simulink model "HDLTxRx"  (R2024a)
settings: Solver=FixedStepDiscrete  StartTime=0.0  StopTime=stopTime  RelTol=1e-3
values from neighbouring files (symbols this model uses):
  msgQtty = length(msgIn)    [testTxRx.m]
  pWords = [pWords binl2str(pBits{i})]    [testTxRx.m]
undefined symbols (not defined in the file or in its folder): CONST
libraries: dspsrcs4 x7, HDL_ieee_8021513 x6, hdlsllib x3
settings Model: DataTypeOverride=Off  SimulationMode=accelerator  Creator=cotti  LastModifiedBy=cotti
settings OptimizationCC: BlockReduction=off  ConditionallyExecuteInputs=off  DefaultParameterBehavior=Inlined  InheritOutputTypeSmallerThanSingle=on
settings DebuggingCC: ArtificialAlgebraicLoopMsg=error  SingleTaskRateTransMsg=error
settings HardwareCC: ProdBitPerPointer=32  ProdBitPerSizeT=32  ProdBitPerPtrDiffT=32  ProdLargestAtomicFloat=None  ProdIntDivRoundTo=Undefined  ProdEndianess=Unspecified  ProdWordSize=32  ProdHWDeviceType=ASIC/FPGA->ASIC/FPGA  TargetBitPerLong=64  TargetBitPerPointer=64  TargetBitPerSizeT=64  TargetBitPerPtrDiffT=64  TargetLongLongMode=on  TargetIntDivRoundTo=Zero  TargetEndianess=LittleEndian  TargetWordSize=64  TargetHWDeviceType=Custom Processor->MATLAB Host Computer  ProdEqTarget=off

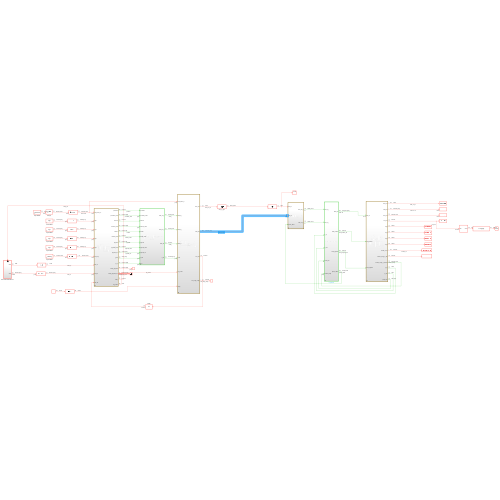
[thumbnail: Simulink's stored preview of the top-level diagram]
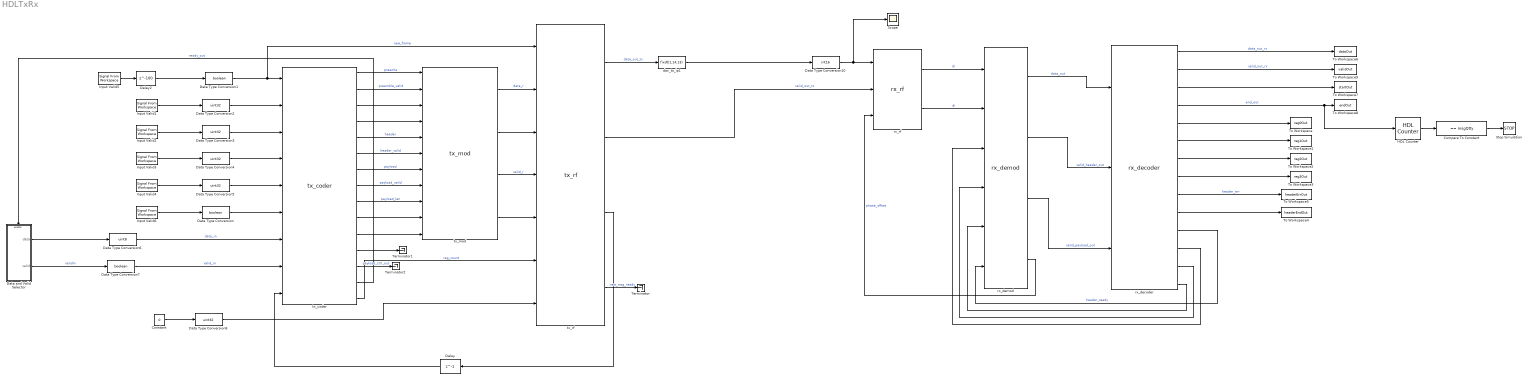
== system HDLTxRx ==
  Compare To Constant : hdlsllib/Logic and Bit Operations/Compare To Constant  relop===  const=msgQtty  OutDataTypeStr=boolean
  Constant : Constant  Value=0  OutDataTypeStr=uint32  SampleTime=-1
  Data Type Conversion : DataTypeConversion  OutDataTypeStr=boolean  SaturateOnIntegerOverflow=off  RndMeth=Floor
  Data Type Conversion1 : DataTypeConversion  OutDataTypeStr=boolean  SaturateOnIntegerOverflow=off  RndMeth=Floor
  Data Type Conversion10 : DataTypeConversion  OutDataTypeStr=int16  ConvertRealWorld=Stored Integer (SI)  SaturateOnIntegerOverflow=off  RndMeth=Floor
  Data Type Conversion{2..5,8} (5 alike) : DataTypeConversion  OutDataTypeStr=uint32  SaturateOnIntegerOverflow=off  RndMeth=Floor
  Data Type Conversion6 : DataTypeConversion  OutDataTypeStr=uint8  SaturateOnIntegerOverflow=off  RndMeth=Floor
  Data Type Conversion7 : DataTypeConversion  OutDataTypeStr=boolean  SaturateOnIntegerOverflow=off  RndMeth=Floor
  Data and Valid Selector : Subsystem  TreatAsAtomicUnit=on
  Delay : Delay  DelayLength=1  InitialCondition=0  UseCircularBuffer=on
  Delay2 : Delay  DelayLength=100  InitialCondition=0  UseCircularBuffer=on
  HDL Counter : hdlsllib/Sources/HDL Counter  CountType=Free running  CountInit=0  CountStep=1  CountMax=25  CountFromType=Initial value  CountFrom=0  CountResetPort=off  CountLoadPort=off  CountEnbPort=on  CountDirPort=off  CountHitOutputPort=off  CountDataType=Unsigned  CountWordLen=32  CountFracLen=0  CountSampTime=1
  Input Valid1 : dspsrcs4/Signal From Workspace  X=reg0  Ts=1/CONST.fs  nsamps=1  OutputAfterFinalValue=Setting to zero  ignoreOrWarnInputAndFrameLengths=off  OutputFrames=off
  Input Valid2 : dspsrcs4/Signal From Workspace  X=reg1  Ts=1/CONST.fs  nsamps=1  OutputAfterFinalValue=Setting to zero  ignoreOrWarnInputAndFrameLengths=off  OutputFrames=off
  Input Valid3 : dspsrcs4/Signal From Workspace  X=reg2  Ts=1/CONST.fs  nsamps=1  OutputAfterFinalValue=Setting to zero  ignoreOrWarnInputAndFrameLengths=off  OutputFrames=off
  Input Valid4 : dspsrcs4/Signal From Workspace  X=reg3  Ts=1/CONST.fs  nsamps=1  OutputAfterFinalValue=Setting to zero  ignoreOrWarnInputAndFrameLengths=off  OutputFrames=off
  Input Valid5 : dspsrcs4/Signal From Workspace  X=newFrame  Ts=1/CONST.fs  nsamps=1  OutputAfterFinalValue=Setting to zero  ignoreOrWarnInputAndFrameLengths=off  OutputFrames=off
  Input Valid6 : dspsrcs4/Signal From Workspace  X=validReg  Ts=1/CONST.fs  nsamps=1  OutputAfterFinalValue=Setting to zero  ignoreOrWarnInputAndFrameLengths=off  OutputFrames=off
  Scope : Scope
  Stop Simulation : Stop
  Terminator : Terminator
  Terminator1 : Terminator
  Terminator2 : Terminator
  To Workspace : ToWorkspace  VariableName=reg0Out  SampleTime=1/CONST.fs
      settings: Save2DSignal=2-D array (concatenate along first dimension)
  To Workspace1 : ToWorkspace  VariableName=reg1Out  SampleTime=1/CONST.fs
      settings: Save2DSignal=2-D array (concatenate along first dimension)
  To Workspace2 : ToWorkspace  VariableName=reg2Out  SampleTime=1/CONST.fs
      settings: Save2DSignal=2-D array (concatenate along first dimension)
  To Workspace3 : ToWorkspace  VariableName=reg3Out  SampleTime=1/CONST.fs
      settings: Save2DSignal=2-D array (concatenate along first dimension)
  To Workspace4 : ToWorkspace  VariableName=headerEndOut  SampleTime=1/CONST.fs
      settings: Save2DSignal=2-D array (concatenate along first dimension)
  To Workspace5 : ToWorkspace  VariableName=headerErrOut  SampleTime=1/CONST.fs
      settings: Save2DSignal=2-D array (concatenate along first dimension)
  To Workspace6 : ToWorkspace  VariableName=dataOut  SampleTime=1/CONST.fs
      settings: Save2DSignal=2-D array (concatenate along first dimension)
  To Workspace7 : ToWorkspace  VariableName=startOut  SampleTime=1/CONST.fs
      settings: Save2DSignal=2-D array (concatenate along first dimension)
  To Workspace8 : ToWorkspace  VariableName=endOut  SampleTime=1/CONST.fs
      settings: Save2DSignal=2-D array (concatenate along first dimension)
  To Workspace9 : ToWorkspace  VariableName=validOut  SampleTime=1/CONST.fs
      settings: Save2DSignal=2-D array (concatenate along first dimension)
  dac_to_ip1 : DataTypeConversion  OutDataTypeStr=fixdt(1,14,13)  ConvertRealWorld=Stored Integer (SI)  SaturateOnIntegerOverflow=off  RndMeth=Floor
  rx_decoder : HDL_ieee_8021513/rx_decoder  SystemSampleTime=-1  VariantActivationTime=update diagram  AllowFlexibleInterface=on  Latency=0  AutoFrameSizeCalculation=off
      settings: SourceProductName=HDL IEEE 8021513
  rx_demod : HDL_ieee_8021513/rx_demod  SystemSampleTime=-1  VariantActivationTime=update diagram  AllowFlexibleInterface=on  Latency=0  AutoFrameSizeCalculation=off
      settings: SourceProductName=HDL IEEE 8021513
  rx_rf : HDL_ieee_8021513/rx_rf  SystemSampleTime=-1  VariantActivationTime=update diagram  AllowFlexibleInterface=on  Latency=0  AutoFrameSizeCalculation=off
      settings: SourceProductName=HDL IEEE 8021513
  tx_coder : HDL_ieee_8021513/tx_coder  SystemSampleTime=-1  VariantActivationTime=update diagram  AllowFlexibleInterface=on  Latency=0  AutoFrameSizeCalculation=off
      settings: SourceProductName=HDL IEEE 8021513
  tx_mod : HDL_ieee_8021513/tx_mod  SystemSampleTime=-1  VariantActivationTime=update diagram  AllowFlexibleInterface=on  Latency=0  AutoFrameSizeCalculation=off
      settings: SourceProductName=HDL IEEE 8021513
  tx_rf : HDL_ieee_8021513/tx_rf  SystemSampleTime=-1  VariantActivationTime=update diagram  AllowFlexibleInterface=on  Latency=0  AutoFrameSizeCalculation=off
      settings: SourceProductName=HDL IEEE 8021513
  wires:
  tx_mod/1 -> tx_rf/2  "data_r"
  tx_coder/1 -> tx_mod/1  "preamle"
  tx_mod/4 -> tx_rf/5
  Data and Valid Selector/2(valid) -> Data Type Conversion7/1  "validIn"
  tx_coder/7 -> tx_mod/7  "payload"
  Input Valid5/1 -> Delay2/1
  Input Valid2/1 -> Data Type Conversion3/1
  tx_coder/6 -> tx_mod/6  "header_valid"
  tx_coder/3 -> tx_mod/3
  tx_coder/8 -> tx_mod/8  "payload_valid"
  tx_coder/15 -> tx_rf/6  "reg_count"
  tx_rf/1 -> dac_to_ip1/1  "data_out_tx"
  tx_coder/4 -> tx_mod/4
  Data Type Conversion/1 -> tx_coder/6
  tx_mod/2 -> tx_rf/3
  Data Type Conversion7/1 -> tx_coder/8  "valid_in"
  Data Type Conversion6/1 -> tx_coder/7  "data_in"
  tx_coder/5 -> tx_mod/5  "header"
  Input Valid4/1 -> Data Type Conversion5/1
  Data and Valid Selector/1(data) -> Data Type Conversion6/1
  tx_coder/9 -> tx_mod/9  "payload_len"
  Input Valid6/1 -> Data Type Conversion/1
  Data Type Conversion1/1 -> tx_coder/1, tx_rf/1  "new_frame"
  tx_coder/14 -> Data and Valid Selector/Enable  "ready_out"
  tx_coder/10 -> tx_mod/10
  tx_mod/3 -> tx_rf/4  "valid_r"
  tx_coder/11 -> tx_mod/11
  tx_rf/3 -> Delay/1
  Delay2/1 -> Data Type Conversion1/1
  Data Type Conversion2/1 -> tx_coder/2
  Data Type Conversion8/1 -> tx_rf/7
  tx_coder/2 -> tx_mod/2  "preamble_valid"
  Input Valid3/1 -> Data Type Conversion4/1
  Input Valid1/1 -> Data Type Conversion2/1
  Data Type Conversion4/1 -> tx_coder/4
  Data Type Conversion3/1 -> tx_coder/3
  Delay/1 -> tx_coder/9
  Data Type Conversion5/1 -> tx_coder/5
  Constant/1 -> Data Type Conversion8/1
  tx_rf/4 -> Terminator/1  "new_msg_ready"
  tx_coder/12 -> Terminator1/1
  tx_coder/13 -> Terminator2/1  "payload_ctrl_out"
  HDL Counter/1 -> Compare To Constant/1
  rx_rf/1 -> rx_demod/1  "dr"
  rx_decoder/8 -> To Workspace3/1
  rx_decoder/5 -> To Workspace/1
  Compare To Constant/1 -> Stop Simulation/1
  rx_demod/2 -> rx_decoder/2  "valid_header_out"
  rx_demod/4 -> rx_rf/3  "phase_offset"
  rx_decoder/2 -> To Workspace9/1  "valid_out_rx"
  dac_to_ip1/1 -> Data Type Conversion10/1
  rx_decoder/4 -> HDL Counter/1, To Workspace8/1  "end_out"
  rx_decoder/12 -> rx_demod/3
  rx_decoder/13 -> rx_demod/4
  rx_decoder/10 -> To Workspace4/1
  rx_decoder/3 -> To Workspace7/1
  rx_decoder/9 -> To Workspace5/1  "header_err"
  rx_decoder/14 -> rx_demod/5
  rx_decoder/7 -> To Workspace2/1
  rx_decoder/6 -> To Workspace1/1
  Data Type Conversion10/1 -> Scope/1, rx_rf/1
  rx_demod/1 -> rx_decoder/1  "data_out"
  tx_rf/2 -> rx_rf/2  "valid_out_tx"
  rx_demod/3 -> rx_decoder/3  "valid_payload_out"
  rx_rf/2 -> rx_demod/2  "di"
  rx_decoder/1 -> To Workspace6/1  "data_out_rx"
  rx_decoder/11 -> rx_demod/6  "header_ready"

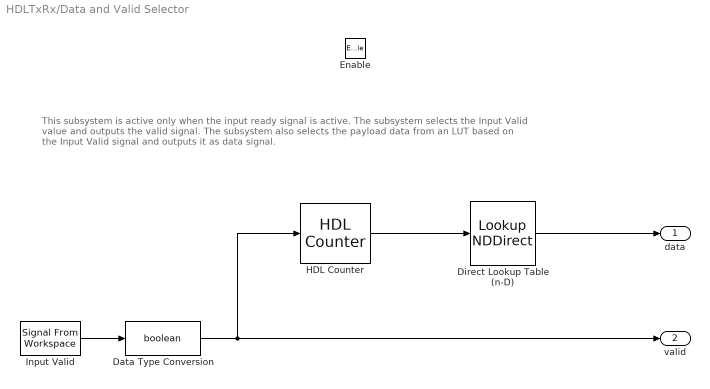
== system HDLTxRx/Data and Valid Selector ==
  note: This subsystem is active only when the input ready signal is active. The subsystem selects the Input Valid value and outputs the valid signal.
      | The subsystem also selects the payload data from an LUT based on the Input Valid signal and outputs it as data signal.
  Enable : EnablePort
  Data Type Conversion : DataTypeConversion  OutDataTypeStr=boolean  SaturateOnIntegerOverflow=off  RndMeth=Floor
  Direct Lookup Table (n-D) : LookupNDDirect  NumberOfTableDimensions=1  Table=uint8(pWords')  DiagnosticForOutOfRangeInput=Error  TableDataTypeStr=uint8
  HDL Counter : hdlsllib/Sources/HDL Counter  CountType=Count limited  CountInit=0  CountStep=1  CountMax=length(pWords) -1  CountFromType=Initial value  CountFrom=0  CountResetPort=off  CountLoadPort=off  CountEnbPort=on  CountDirPort=off  CountHitOutputPort=off  CountDataType=Unsigned  CountWordLen=nextpow2(length(pWords))  CountFracLen=0  CountSampTime=1
  Input Valid : dspsrcs4/Signal From Workspace  X=validIn  Ts=1/CONST.fs  nsamps=1  OutputAfterFinalValue=Setting to zero  ignoreOrWarnInputAndFrameLengths=off  OutputFrames=off
  data : Outport  InitialOutput=0  VectorParamsAs1DForOutWhenUnconnected=off
  valid : Outport  Port=2  InitialOutput=0  VectorParamsAs1DForOutWhenUnconnected=off
  wires:
  HDL Counter/1 -> Direct Lookup Table (n-D)/1
  Direct Lookup Table (n-D)/1 -> data/1
  Input Valid/1 -> Data Type Conversion/1
  Data Type Conversion/1 -> valid/1, HDL Counter/1
